simulink model "test_master_task"  (Simulink 3.00)
libraries: mathlib x10, inoutlib x2, arclib x1

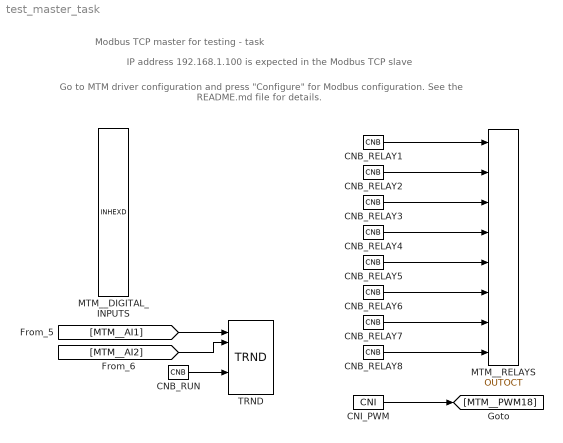
== system test_master_task ==
  note: IP address 192.168.1.100 is expected in the Modbus TCP slave
  note: Go to MTM driver configuration and press "Configure" for Modbus configuration.
      |
      | See the README.md file for details.
  note: Modbus TCP master for testing - task
  CNB_RELAY{1,3,5,7} (4 alike) : mathlib/CNB  YCN=off
  CNB_RELAY{2,4,6,8} (4 alike) : mathlib/CNB  YCN=on
  CNB_RUN : mathlib/CNB  YCN=on
  CNI_PWM : mathlib/CNI  icn=512
  MTM__DIGITAL_INPUTS : inoutlib/INHEXD
  MTM__RELAYS : inoutlib/OUTOCT
  TRND : arclib/TRND  n=4  l=1000  btype=8: Double  ptype1=1: Store  ptype2=1: Store  ptype3=1: Store  ptype4=1: Store  pfac=1  afac=0  arc=0  id=1  Title=Trend Title  timesrc=1
  wires:
  CNB_RELAY1/1 -> MTM__RELAYS/1
  CNB_RELAY2/1 -> MTM__RELAYS/2
  CNB_RELAY3/1 -> MTM__RELAYS/3
  CNB_RELAY4/1 -> MTM__RELAYS/4
  CNB_RELAY5/1 -> MTM__RELAYS/5
  CNB_RELAY6/1 -> MTM__RELAYS/6
  CNB_RELAY7/1 -> MTM__RELAYS/7
  CNB_RELAY8/1 -> MTM__RELAYS/8
  CNB_RUN/1 -> TRND/5
  CNI_PWM/1 -> [MTM__PWM18]
  [MTM__AI1] -> TRND/1
  [MTM__AI2] -> TRND/2
